simulink model "state_feedback"  (R2020b)
settings: Solver=VariableStepAuto  StartTime=0.0  StopTime=10  RelTol=1e-3
undefined symbols (not defined in the file or in its folder): K1, K2, K3
settings Model: Creator=Hirsa  LastModifiedBy=Hirsa

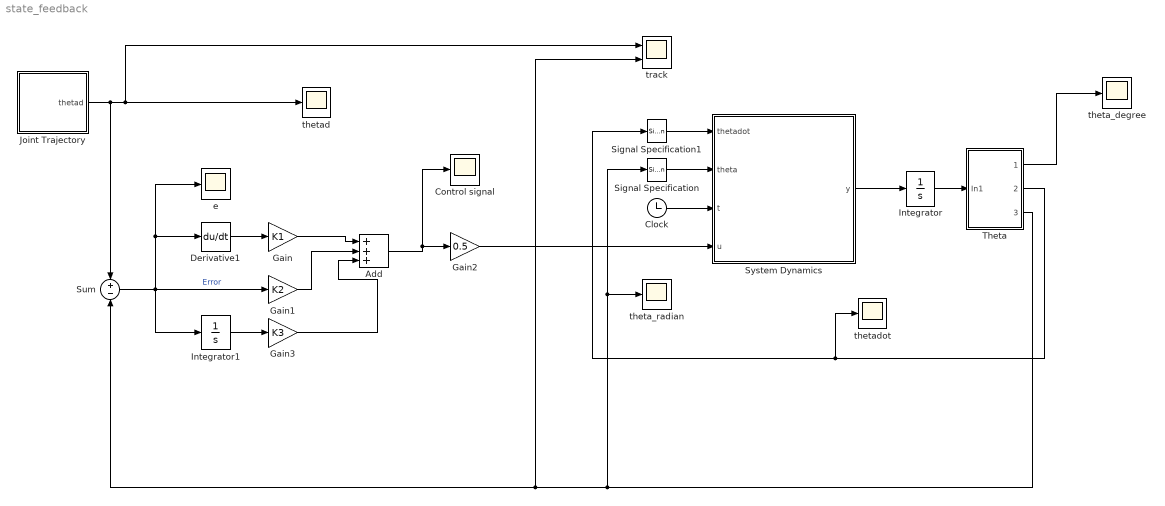
== system state_feedback ==
  Add : Sum  Inputs=+++
  Clock : Clock
  Control signal : Scope
  Derivative1 : Derivative
  Gain : Gain  Gain=K1
  Gain1 : Gain  Gain=K2
  Gain2 : Gain  Gain=0.5
  Gain3 : Gain  Gain=K3
  Integrator : Integrator  InitialCondition=[0;0;0;0;0;0 ;zeros(6,1)]  UpperSaturationLimit=10000  LowerSaturationLimit=-10000  AbsoluteTolerance=-1
  Integrator1 : Integrator  InitialCondition=[0;0;0;0;0;0]  UpperSaturationLimit=10000  LowerSaturationLimit=-10000  AbsoluteTolerance=-1
  Joint Trajectory : Subsystem
  Signal Specification : SignalSpecification  Dimensions=6
  Signal Specification1 : SignalSpecification  Dimensions=6
  Sum : Sum  Inputs=+|-
  System Dynamics : MATLAB Function  TreatAsAtomicUnit=on
  Theta : Subsystem
  e : Scope
  theta_degree : Scope
  theta_radian : Scope
  thetad : Scope
  thetadot : Scope
  track : Scope  NumInputPorts=2
  wires:
  Joint Trajectory/1(thetad) -> Sum/1, thetad/1, track/1
  Theta/3(Theta Radian) -> track/2, Sum/2, theta_radian/1, Signal Specification/1
  Sum/1 -> Integrator1/1, Gain1/1, Derivative1/1, e/1  "Error"
  Clock/1 -> System Dynamics/3(t)
  Gain/1 -> Add/1
  Derivative1/1 -> Gain/1
  Add/1 -> Gain2/1, Control signal/1
  Theta/1(Theta Degree) -> theta_degree/1
  System Dynamics/1(y) -> Integrator/1
  Integrator/1 -> Theta/1(In1)
  Signal Specification/1 -> System Dynamics/2(theta)
  Signal Specification1/1 -> System Dynamics/1(thetadot)
  Theta/2(thetadot) -> Signal Specification1/1, thetadot/1
  Gain2/1 -> System Dynamics/4(u)
  Gain1/1 -> Add/2
  Gain3/1 -> Add/3
  Integrator1/1 -> Gain3/1

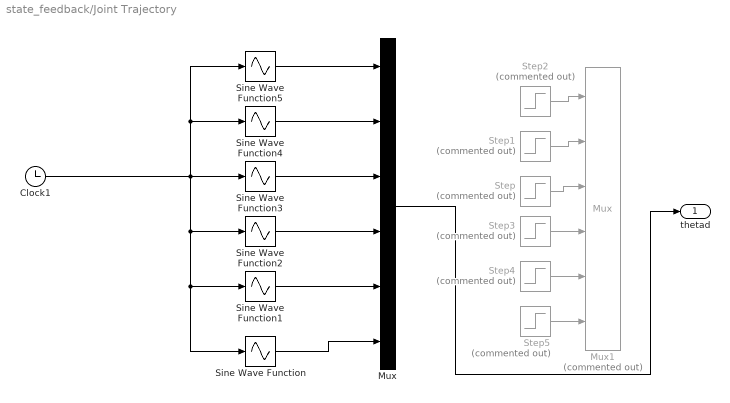
== system state_feedback/Joint Trajectory ==
  Clock1 : Clock
  Mux : Mux  Inputs=6
  Mux1 : Mux  Commented=on  Inputs=6
  Sine Wave Function : Sin  TimeSource=Use external signal  Bias=3  Frequency=0.3  SampleTime=0
  Sine Wave Function1 : Sin  TimeSource=Use external signal  Bias=0.1  Frequency=0.1  SampleTime=0
  Sine Wave Function2 : Sin  TimeSource=Use external signal  Frequency=0.4  SampleTime=0
  Sine Wave Function3 : Sin  TimeSource=Use external signal  Bias=1  SampleTime=0
  Sine Wave Function4 : Sin  TimeSource=Use external signal  Bias=-1  Frequency=1/6  SampleTime=0
  Sine Wave Function5 : Sin  TimeSource=Use external signal  Bias=-1  Frequency=1/5  SampleTime=0
  Step : Step  Commented=on  Time=0  After=-5  SampleTime=0
  Step1 : Step  Commented=on  Time=0  After=-5  SampleTime=0
  Step2 : Step  Commented=on  Time=0  After=-1  SampleTime=0
  Step3 : Step  Commented=on  Time=0  After=5  SampleTime=0
  Step4 : Step  Commented=on  Time=0  After=5  SampleTime=0
  Step5 : Step  Commented=on  Time=0  After=5  SampleTime=0
  thetad : Outport
  wires:
  Clock1/1 -> Sine Wave Function5/1, Sine Wave Function4/1, Sine Wave Function1/1, Sine Wave Function/1, Sine Wave Function2/1, Sine Wave Function3/1
  Step3/1 -> Mux1/4
  Step4/1 -> Mux1/5
  Step5/1 -> Mux1/6
  Step2/1 -> Mux1/1
  Step1/1 -> Mux1/2
  Step/1 -> Mux1/3
  Mux/1 -> thetad/1
  Sine Wave Function5/1 -> Mux/1
  Sine Wave Function4/1 -> Mux/2
  Sine Wave Function3/1 -> Mux/3
  Sine Wave Function2/1 -> Mux/4
  Sine Wave Function1/1 -> Mux/5
  Sine Wave Function/1 -> Mux/6

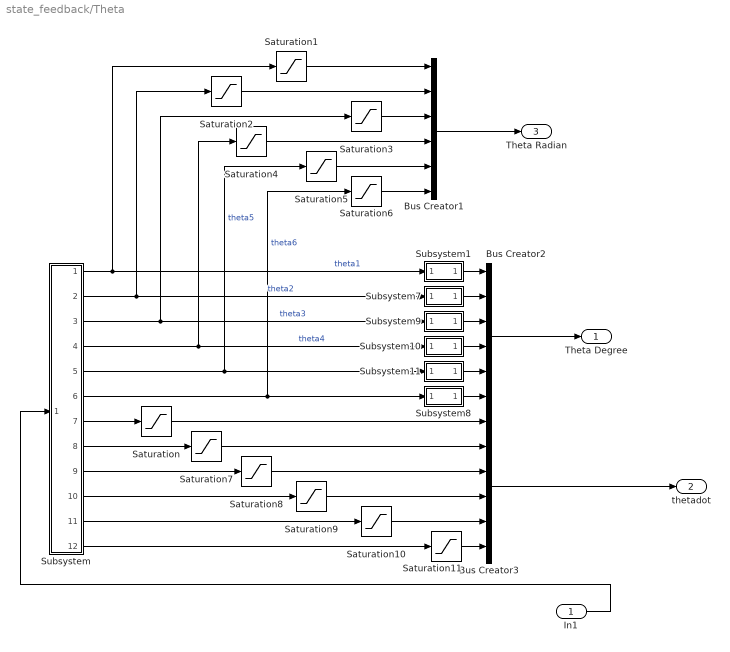
== system state_feedback/Theta ==
  In1 : Inport
  Bus Creator1 : BusCreator  Inputs=6
  Bus Creator2 : BusCreator  Inputs=6
  Bus Creator3 : BusCreator  Inputs=6
  Saturation : Saturate  UpperLimit=2.23  LowerLimit=-2.23
  Saturation1 : Saturate  UpperLimit=deg2rad(185)  LowerLimit=deg2rad(-185)
  Saturation10 : Saturate  UpperLimit=4.28  LowerLimit=-4.28
  Saturation11 : Saturate  UpperLimit=5.62  LowerLimit=-5.62
  Saturation2 : Saturate  UpperLimit=deg2rad(135)  LowerLimit=deg2rad(-135)
  Saturation3 : Saturate  UpperLimit=deg2rad(150)  LowerLimit=deg2rad(-150)
  Saturation4 : Saturate  UpperLimit=deg2rad(350)  LowerLimit=deg2rad(-350)
  Saturation5 : Saturate  UpperLimit=deg2rad(119)  LowerLimit=deg2rad(-119)
  Saturation6 : Saturate  UpperLimit=deg2rad(350)  LowerLimit=deg2rad(-350)
  Saturation7 : Saturate  UpperLimit=1.78  LowerLimit=-1.78
  Saturation8 : Saturate  UpperLimit=2.23  LowerLimit=-2.23
  Saturation9 : Saturate  UpperLimit=4.54  LowerLimit=-4.54
  Subsystem : Subsystem
  Subsystem1 : Subsystem
  Subsystem10 : Subsystem
  Subsystem11 : Subsystem
  Subsystem7 : Subsystem
  Subsystem8 : Subsystem
  Subsystem9 : Subsystem
  Theta Degree : Outport
  thetadot : Outport  Port=2
  Theta Radian : Outport  Port=3
  wires:
  In1/1 -> Subsystem/1(In1)
  Subsystem/11(Out11) -> Saturation10/1
  Subsystem/9(Out9) -> Saturation8/1
  Subsystem/12(Out12) -> Saturation11/1
  Subsystem/10(Out10) -> Saturation9/1
  Subsystem/8(Out8) -> Saturation7/1
  Subsystem/7(Out7) -> Saturation/1
  Subsystem7/1(Out1) -> Bus Creator2/2
  Subsystem1/1(Out1) -> Bus Creator2/1
  Subsystem8/1(Out1) -> Bus Creator2/6
  Subsystem9/1(Out1) -> Bus Creator2/3
  Subsystem10/1(Out1) -> Bus Creator2/4
  Subsystem11/1(Out1) -> Bus Creator2/5
  Subsystem/1(Out1) -> Saturation1/1, Subsystem1/1(In1)  "theta1"
  Subsystem/3(Out3) -> Subsystem9/1(In1), Saturation3/1  "theta3"
  Subsystem/4(Out4) -> Subsystem10/1(In1), Saturation4/1  "theta4"
  Subsystem/6(Out6) -> Subsystem8/1(In1), Saturation6/1  "theta6"
  Subsystem/5(Out5) -> Subsystem11/1(In1), Saturation5/1  "theta5"
  Subsystem/2(Out2) -> Subsystem7/1(In1), Saturation2/1  "theta2"
  Bus Creator1/1 -> Theta Radian/1
  Bus Creator2/1 -> Theta Degree/1
  Bus Creator3/1 -> thetadot/1
  Saturation1/1 -> Bus Creator1/1
  Saturation6/1 -> Bus Creator1/6
  Saturation5/1 -> Bus Creator1/5
  Saturation4/1 -> Bus Creator1/4
  Saturation3/1 -> Bus Creator1/3
  Saturation2/1 -> Bus Creator1/2
  Saturation11/1 -> Bus Creator3/6
  Saturation10/1 -> Bus Creator3/5
  Saturation9/1 -> Bus Creator3/4
  Saturation8/1 -> Bus Creator3/3
  Saturation7/1 -> Bus Creator3/2
  Saturation/1 -> Bus Creator3/1

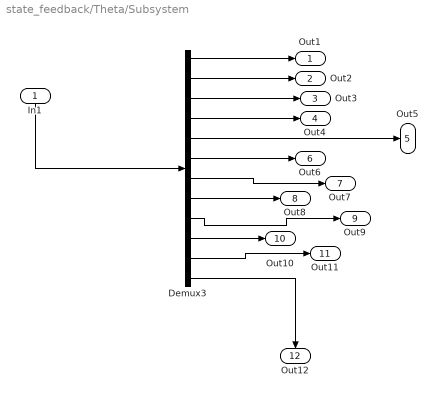
== system state_feedback/Theta/Subsystem ==
  In1 : Inport
  Demux3 : Demux  Outputs=12
  Out1 : Outport
  Out2 : Outport  Port=2
  Out3 : Outport  Port=3
  Out4 : Outport  Port=4
  Out5 : Outport  Port=5
  Out6 : Outport  Port=6
  Out7 : Outport  Port=7
  Out8 : Outport  Port=8
  Out9 : Outport  Port=9
  Out10 : Outport  Port=10
  Out11 : Outport  Port=11
  Out12 : Outport  Port=12
  wires:
  Demux3/1 -> Out1/1
  Demux3/9 -> Out9/1
  Demux3/10 -> Out10/1
  Demux3/7 -> Out7/1
  In1/1 -> Demux3/1
  Demux3/8 -> Out8/1
  Demux3/11 -> Out11/1
  Demux3/5 -> Out5/1
  Demux3/3 -> Out3/1
  Demux3/2 -> Out2/1
  Demux3/4 -> Out4/1
  Demux3/6 -> Out6/1
  Demux3/12 -> Out12/1

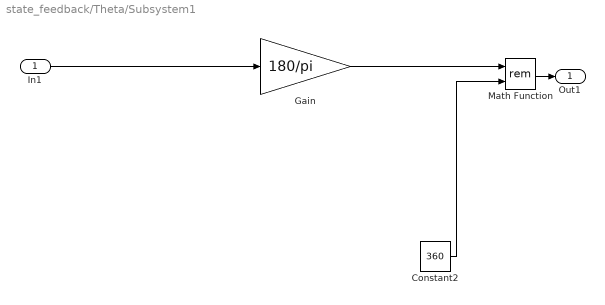
== system state_feedback/Theta/Subsystem1 ==
  In1 : Inport
  Constant2 : Constant  Value=360
  Gain : Gain  Gain=180/pi
  Math Function : Math  Operator=rem  SignedPower=on  SaturateOnIntegerOverflow=on
  Out1 : Outport
  wires:
  Math Function/1 -> Out1/1
  In1/1 -> Gain/1
  Constant2/1 -> Math Function/2
  Gain/1 -> Math Function/1

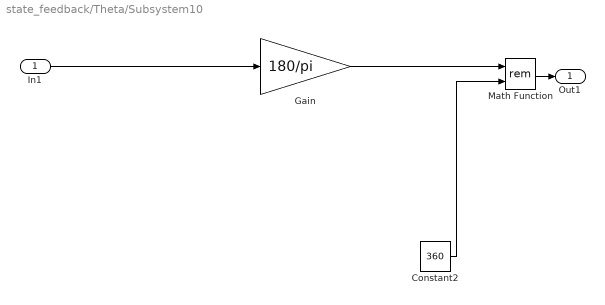
== system state_feedback/Theta/Subsystem10 ==
  In1 : Inport
  Constant2 : Constant  Value=360
  Gain : Gain  Gain=180/pi
  Math Function : Math  Operator=rem  SignedPower=on  SaturateOnIntegerOverflow=on
  Out1 : Outport
  wires:
  Math Function/1 -> Out1/1
  In1/1 -> Gain/1
  Constant2/1 -> Math Function/2
  Gain/1 -> Math Function/1

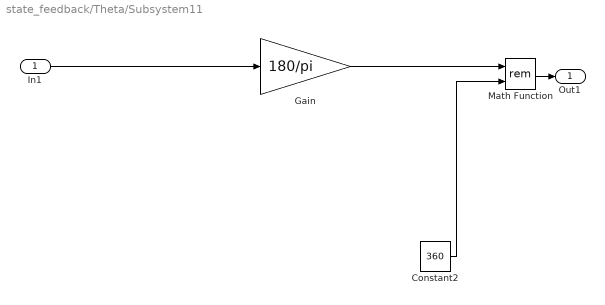
== system state_feedback/Theta/Subsystem11 ==
  In1 : Inport
  Constant2 : Constant  Value=360
  Gain : Gain  Gain=180/pi
  Math Function : Math  Operator=rem  SignedPower=on  SaturateOnIntegerOverflow=on
  Out1 : Outport
  wires:
  Math Function/1 -> Out1/1
  In1/1 -> Gain/1
  Constant2/1 -> Math Function/2
  Gain/1 -> Math Function/1

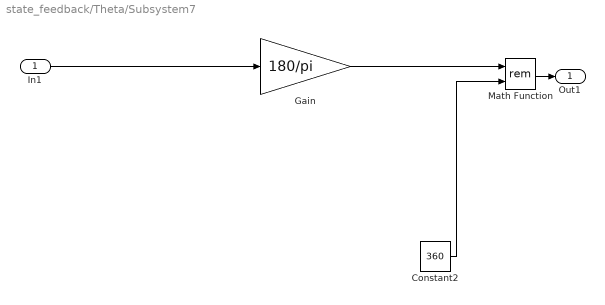
== system state_feedback/Theta/Subsystem7 ==
  In1 : Inport
  Constant2 : Constant  Value=360
  Gain : Gain  Gain=180/pi
  Math Function : Math  Operator=rem  SignedPower=on  SaturateOnIntegerOverflow=on
  Out1 : Outport
  wires:
  Math Function/1 -> Out1/1
  In1/1 -> Gain/1
  Constant2/1 -> Math Function/2
  Gain/1 -> Math Function/1

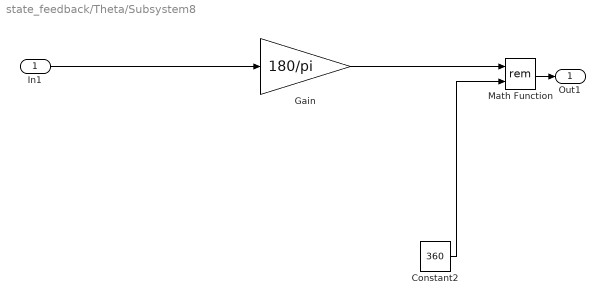
== system state_feedback/Theta/Subsystem8 ==
  In1 : Inport
  Constant2 : Constant  Value=360
  Gain : Gain  Gain=180/pi
  Math Function : Math  Operator=rem  SignedPower=on  SaturateOnIntegerOverflow=on
  Out1 : Outport
  wires:
  Math Function/1 -> Out1/1
  In1/1 -> Gain/1
  Constant2/1 -> Math Function/2
  Gain/1 -> Math Function/1

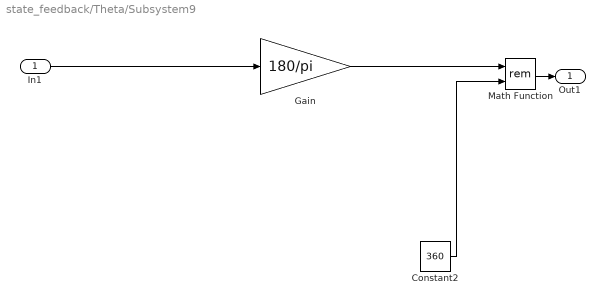
== system state_feedback/Theta/Subsystem9 ==
  In1 : Inport
  Constant2 : Constant  Value=360
  Gain : Gain  Gain=180/pi
  Math Function : Math  Operator=rem  SignedPower=on  SaturateOnIntegerOverflow=on
  Out1 : Outport
  wires:
  Math Function/1 -> Out1/1
  In1/1 -> Gain/1
  Constant2/1 -> Math Function/2
  Gain/1 -> Math Function/1

== matlab function state_feedback/System Dynamics ==
  data: thetadot input; theta input; t input; u input; y output
function y = fcn(thetadot,theta,t,u)

theta1=theta(1)
theta2=theta(2)
theta3=theta(3)
theta4=theta(4)
theta5=theta(5)
theta6=theta(6)

thetadot1=thetadot(1)
thetadot2=thetadot(2)
thetadot3=thetadot(3)
thetadot4=thetadot(4)
thetadot5=thetadot(5)
thetadot6=thetadot(6)


C = [0.52*thetadot1*thetadot2*sin(theta3) + 0.43*thetadot1*thetadot2*sin(2.0*theta2) + 0.59*thetadot1*thetadot2*sin(2.0*theta3) + 0.59*thetadot1*thetadot3*sin(2.0*theta2) + 0.59*thetadot1*thetadot3*sin(2.0*theta3) - 0.0016*thetadot2*thetadot4*sin(theta2)*sin(theta3) - 0.0016*thetadot3*thetadot4*sin(theta2)*sin(theta3) - 1.04*thetadot1*thetadot2*cos(theta2)^2*sin(theta3) - 0.52*thetadot1*thetadot3*cos(theta2)^2*sin(theta3) + 0.0016*thetadot2*thetadot4*cos(theta2)*cos(theta3) + 0.0016*thetadot3*thetadot4*cos(theta2)*cos(theta3) - 2.36*thetadot1*thetadot2*cos(theta2)*cos(theta3)^2*sin(theta2) - 2.36*thetadot1*thetadot2*cos(theta2)^2*cos(theta3)*sin(theta3) - 2.36*thetadot1*thetadot3*cos(theta2)*cos(theta3)^2*sin(theta2) - 2.36*thetadot1*thetadot3*cos(theta2)^2*cos(theta3)*sin(theta3) + (thetadot2*thetadot6*cos(theta2)*cos(theta3)*cos(theta5))/10000 - 0.0006*thetadot4*thetadot5*cos(theta2)*cos(theta3)*cos(theta4) + (thetadot3*thetadot6*cos(theta2)*cos(theta3)*cos(theta5))/10000 - 1.04*thetadot1*thetadot2*cos(theta2)*cos(theta3)*sin(theta2) - 0.52*thetadot1*thetadot3*cos(theta2)*cos(theta3)*sin(theta2) + 0.0006*thetadot2*thetadot5*cos(theta2)*sin(theta3)*sin(theta4) + 0.0006*thetadot2*thetadot5*cos(theta3)*sin(theta2)*sin(theta4) + 0.0006*thetadot3*thetadot5*cos(theta2)*sin(theta3)*sin(theta4) + 0.0006*thetadot3*thetadot5*cos(theta3)*sin(theta2)*sin(theta4) - 0.0001*thetadot2*thetadot6*cos(theta5)*sin(theta2)*sin(theta3) + 0.0006*thetadot4*thetadot5*cos(theta4)*sin(theta2)*sin(theta3) - 0.0001*thetadot3*thetadot6*cos(theta5)*sin(theta2)*sin(theta3) - 0.0001*thetadot5*thetadot6*cos(theta2)*sin(theta3)*sin(theta5) - 0.0001*thetadot5*thetadot6*cos(theta3)*sin(theta2)*sin(theta5) + (thetadot5*thetadot6*cos(theta2)*cos(theta3)*cos(theta4)*cos(theta5))/10000 - 0.0001*thetadot2*thetadot6*cos(theta2)*cos(theta4)*sin(theta3)*sin(theta5) - 0.0001*thetadot2*thetadot6*cos(theta3)*cos(theta4)*sin(theta2)*sin(theta5) - 0.0001*thetadot3*thetadot6*cos(theta2)*cos(theta4)*sin(theta3)*sin(theta5) - 0.0001*thetadot3*thetadot6*cos(theta3)*cos(theta4)*sin(theta2)*sin(theta5) - 0.0001*thetadot4*thetadot6*cos(theta2)*cos(theta3)*sin(theta4)*sin(theta5) - 0.0001*thetadot5*thetadot6*cos(theta4)*cos(theta5)*sin(theta2)*sin(theta3) + (thetadot4*thetadot6*sin(theta2)*sin(theta3)*sin(theta4)*sin(theta5))/10000;
                                                                                                                                                                                                                                                                                                                                                                                                                                                                                                                                                                                                                                                                                                                                                                                                                                                                                                                                                                                                                                                                                                                                                                                                                                                                                                            0.52*thetadot1^2*cos(theta2)^2*sin(theta3) - 0.26*thetadot3^2*sin(theta3) - 0.215*thetadot1^2*sin(2.0*theta2) - 0.295*thetadot1^2*sin(2.0*theta3) - 0.52*thetadot2*thetadot3*sin(theta3) - 0.0006*thetadot4*thetadot5*sin(theta4) - 0.26*thetadot1^2*sin(theta3) + 0.0001*thetadot4*thetadot6*cos(theta4)*sin(theta5) + 0.0001*thetadot5*thetadot6*cos(theta5)*sin(theta4) + 0.0016*thetadot1*thetadot4*sin(theta2)*sin(theta3) + 1.18*thetadot1^2*cos(theta2)*cos(theta3)^2*sin(theta2) + 1.18*thetadot1^2*cos(theta2)^2*cos(theta3)*sin(theta3) + 0.52*thetadot1^2*cos(theta2)*cos(theta3)*sin(theta2) - 0.0016*thetadot1*thetadot4*cos(theta2)*cos(theta3) - (thetadot1*thetadot6*cos(theta2)*cos(theta3)*cos(theta5))/10000 - 0.0006*thetadot1*thetadot5*cos(theta2)*sin(theta3)*sin(theta4) - 0.0006*thetadot1*thetadot5*cos(theta3)*sin(theta2)*sin(theta4) + 0.0001*thetadot1*thetadot6*cos(theta5)*sin(theta2)*sin(theta3) + 0.0001*thetadot1*thetadot6*cos(theta2)*cos(theta4)*sin(theta3)*sin(theta5) + 0.0001*thetadot1*thetadot6*cos(theta3)*cos(theta4)*sin(theta2)*sin(theta5);
                                                                                                                                                                                                                                                                                                                                                                                                                                                                                                                                                                                                                                                                                                                                                                                                                                                                                                                                                                                                                                                                                                                                                                                                                                                                                                                                                                                  0.26*thetadot2^2*sin(theta3) - 0.295*thetadot1^2*sin(2.0*theta2) - 0.295*thetadot1^2*sin(2.0*theta3) - 0.0006*thetadot4*thetadot5*sin(theta4) + 0.26*thetadot1^2*cos(theta2)^2*sin(theta3) + 0.0001*thetadot4*thetadot6*cos(theta4)*sin(theta5) + 0.0001*thetadot5*thetadot6*cos(theta5)*sin(theta4) + 0.0016*thetadot1*thetadot4*sin(theta2)*sin(theta3) + 1.18*thetadot1^2*cos(theta2)*cos(theta3)^2*sin(theta2) + 1.18*thetadot1^2*cos(theta2)^2*cos(theta3)*sin(theta3) + 0.26*thetadot1^2*cos(theta2)*cos(theta3)*sin(theta2) - 0.0016*thetadot1*thetadot4*cos(theta2)*cos(theta3) - (thetadot1*thetadot6*cos(theta2)*cos(theta3)*cos(theta5))/10000 - 0.0006*thetadot1*thetadot5*cos(theta2)*sin(theta3)*sin(theta4) - 0.0006*thetadot1*thetadot5*cos(theta3)*sin(theta2)*sin(theta4) + 0.0001*thetadot1*thetadot6*cos(theta5)*sin(theta2)*sin(theta3) + 0.0001*thetadot1*thetadot6*cos(theta2)*cos(theta4)*sin(theta3)*sin(theta5) + 0.0001*thetadot1*thetadot6*cos(theta3)*cos(theta4)*sin(theta2)*sin(theta5);
                                                                                                                                                                                                                                                                                                                                                                                                                                                                                                                                                                                                                                                                                                                                                                                                                                                                                                                                                                                                                                                                                                                                                                                                                                                                                                                                                                                                                                                                                                                                                                                                                                                      0.0006*thetadot2*thetadot5*sin(theta4) + 0.0006*thetadot3*thetadot5*sin(theta4) - 0.0001*thetadot5*thetadot6*sin(theta5) - 0.0001*thetadot2*thetadot6*cos(theta4)*sin(theta5) - 0.0001*thetadot3*thetadot6*cos(theta4)*sin(theta5) - 0.0016*thetadot1*thetadot2*sin(theta2)*sin(theta3) - 0.0016*thetadot1*thetadot3*sin(theta2)*sin(theta3) + 0.0016*thetadot1*thetadot2*cos(theta2)*cos(theta3) + 0.0016*thetadot1*thetadot3*cos(theta2)*cos(theta3) + 0.0006*thetadot1*thetadot5*cos(theta2)*cos(theta3)*cos(theta4) - 0.0006*thetadot1*thetadot5*cos(theta4)*sin(theta2)*sin(theta3) + 0.0001*thetadot1*thetadot6*cos(theta2)*cos(theta3)*sin(theta4)*sin(theta5) - 0.0001*thetadot1*thetadot6*sin(theta2)*sin(theta3)*sin(theta4)*sin(theta5);
                                                                                                                                                                                                                                                                                                                                                                                                                                                                                                                                                                                                                                                                                                                                                                                                                                                                                                                                                                                                                                                                                                                                                                                                                                                                                                                                                                                                                                                                    0.0001*thetadot4*thetadot6*sin(theta5) - 0.0006*thetadot3*thetadot4*sin(theta4) - 0.0006*thetadot2*thetadot4*sin(theta4) - 0.0001*thetadot2*thetadot6*cos(theta5)*sin(theta4) - 0.0001*thetadot3*thetadot6*cos(theta5)*sin(theta4) - 0.0006*thetadot1*thetadot4*cos(theta2)*cos(theta3)*cos(theta4) + 0.0006*thetadot1*thetadot2*cos(theta2)*sin(theta3)*sin(theta4) + 0.0006*thetadot1*thetadot2*cos(theta3)*sin(theta2)*sin(theta4) + 0.0006*thetadot1*thetadot3*cos(theta2)*sin(theta3)*sin(theta4) + 0.0006*thetadot1*thetadot3*cos(theta3)*sin(theta2)*sin(theta4) + 0.0006*thetadot1*thetadot4*cos(theta4)*sin(theta2)*sin(theta3) + 0.0001*thetadot1*thetadot6*cos(theta2)*sin(theta3)*sin(theta5) + 0.0001*thetadot1*thetadot6*cos(theta3)*sin(theta2)*sin(theta5) - 0.0001*thetadot1*thetadot6*cos(theta2)*cos(theta3)*cos(theta4)*cos(theta5) + 0.0001*thetadot1*thetadot6*cos(theta4)*cos(theta5)*sin(theta2)*sin(theta3);
                                                                                                                                                                                                                                                                                                                                                                                                                                                                                                                                                                                                                                                                                                                                                                                                                                                                                                                                                                                                                                                                                                0.0001*thetadot2*thetadot4*cos(theta4)*sin(theta5) - 0.0001*thetadot4*thetadot5*sin(theta5) + 0.0001*thetadot2*thetadot5*cos(theta5)*sin(theta4) + 0.0001*thetadot3*thetadot4*cos(theta4)*sin(theta5) + 0.0001*thetadot3*thetadot5*cos(theta5)*sin(theta4) + 0.0001*thetadot1*thetadot2*cos(theta2)*cos(theta3)*cos(theta5) + 0.0001*thetadot1*thetadot3*cos(theta2)*cos(theta3)*cos(theta5) - 0.0001*thetadot1*thetadot2*cos(theta5)*sin(theta2)*sin(theta3) - 0.0001*thetadot1*thetadot3*cos(theta5)*sin(theta2)*sin(theta3) - 0.0001*thetadot1*thetadot5*cos(theta2)*sin(theta3)*sin(theta5) - 0.0001*thetadot1*thetadot5*cos(theta3)*sin(theta2)*sin(theta5) + 0.0001*thetadot1*thetadot5*cos(theta2)*cos(theta3)*cos(theta4)*cos(theta5) - 0.0001*thetadot1*thetadot2*cos(theta2)*cos(theta4)*sin(theta3)*sin(theta5) - 0.0001*thetadot1*thetadot2*cos(theta3)*cos(theta4)*sin(theta2)*sin(theta5) - 0.0001*thetadot1*thetadot3*cos(theta2)*cos(theta4)*sin(theta3)*sin(theta5) - 0.0001*thetadot1*thetadot3*cos(theta3)*cos(theta4)*sin(theta2)*sin(theta5) - 0.0001*thetadot1*thetadot4*cos(theta2)*cos(theta3)*sin(theta4)*sin(theta5) - 0.0001*thetadot1*thetadot5*cos(theta4)*cos(theta5)*sin(theta2)*sin(theta3) + 0.0001*thetadot1*thetadot4*sin(theta2)*sin(theta3)*sin(theta4)*sin(theta5)]
g = [                                           0;
- 12.753*cos(theta2 + theta3) - 7.848*cos(theta2);
                     -12.753*cos(theta2 + theta3);
                                                0;
                                                0;
                                                0]
 
MM = [                                                                                            0.26*cos(2*theta2 + theta3) + 0.08*cos(2*theta2) + 0.295*cos(2*theta2 + 2*theta3) + 0.26*cos(theta3) + 0.6766,                                                                                                                                                                                                                 0,                                                                                                                                                                                                                 0, 0.0016*sin(theta2 + theta3), -0.0006*cos(theta2 + theta3)*sin(theta4), 0.0001*cos(theta2)*cos(theta5)*sin(theta3) + 0.0001*cos(theta3)*cos(theta5)*sin(theta2) + 0.0001*cos(theta2)*cos(theta3)*cos(theta4)*sin(theta5) - 0.0001*cos(theta4)*sin(theta2)*sin(theta3)*sin(theta5);
                                                                                                                                                                                                        0, 7.8248506247897785240381059930909e-42*cos(2.0*theta5) - 3.0783724664287581414052491485713e-41*cos(2.0*theta4) + 0.52*cos(theta3) + 7.8248506247897785240381059930909e-42*cos(2.0*theta4)*cos(2.0*theta5) + 0.9516, 7.8248506247897785240381059930909e-42*cos(2.0*theta5) - 3.0783724664287581414052491485713e-41*cos(2.0*theta4) + 0.26*cos(theta3) + 7.8248506247897785240381059930909e-42*cos(2.0*theta4)*cos(2.0*theta5) + 0.6916,                           0,                       0.0006*cos(theta4),                                                                                                                                                                            0.0001*sin(theta4)*sin(theta5);
                                                                                                                                                                                                       0, 7.8248506247897785240381059930909e-42*cos(2.0*theta5) - 3.0783724664287581414052491485713e-41*cos(2.0*theta4) + 0.26*cos(theta3) + 7.8248506247897785240381059930909e-42*cos(2.0*theta4)*cos(2.0*theta5) + 0.6916,                    1.5134023414708024365976279499531e-41*cos(2.0*theta4) - 3.6545863949591229209690867532201e-42*cos(2.0*theta5) - 1.1479437019748901445007192746311e-41*cos(2.0*theta4)*cos(2.0*theta5) + 0.6916,                           0,                       0.0006*cos(theta4),                                                                                                                                                                            0.0001*sin(theta4)*sin(theta5);
                                                                                                                                                                              0.0016*sin(theta2 + theta3),                                                                                                                                                                                                                 0,                                                                                                                                                                                                                 0,                      0.0016,                                        0,                                                                                                                                                                                        0.0001*cos(theta5);
                                                                                                                                                                 -0.0006*cos(theta2 + theta3)*sin(theta4),                                                                                                                                                                                                0.0006*cos(theta4),                                                                                                                                                                                                0.0006*cos(theta4),                           0,                                   0.0006,                                                                                                                                                                                                         0;
0.0001*cos(theta2)*cos(theta5)*sin(theta3) + 0.0001*cos(theta3)*cos(theta5)*sin(theta2) + 0.0001*cos(theta2)*cos(theta3)*cos(theta4)*sin(theta5) - 0.0001*cos(theta4)*sin(theta2)*sin(theta3)*sin(theta5),                                                                                                                                                                                    0.0001*sin(theta4)*sin(theta5),                                                                                                                                                                                    0.0001*sin(theta4)*sin(theta5),          0.0001*cos(theta5),                                        0,                                                                                                                                                                                                    0.0001]
 
% Fc=[0.002*sign(thetadot1);
%     0.002*sign(thetadot2);
%     0.002*sign(thetadot3);
%     0.002*sign(thetadot4);
%     0.002*sign(thetadot5);
%     0.002*sign(thetadot6)];

Fv=[0.001*(thetadot1);
    0.001*(thetadot2);
    0.001*(thetadot3);
    0.001*(thetadot4);
    0.001*(thetadot5);
    0.001*(thetadot6)];

x=[theta;thetadot]
dx=zeros(12,1)
dx(1)=x(7)
dx(2)=x(8)
dx(3)=x(9)
dx(4)=x(10)
dx(5)=x(11)
dx(6)=x(12)

dx(7:12)=(u)-inv(MM)*(Fv)
y=[dx(1);dx(2);dx(3);dx(4);dx(5);dx(6);dx(7);dx(8);dx(9);dx(10);dx(11);dx(12)]
